simulink model "lab4"  (R2016b)
settings: Solver=VariableStepAuto  StartTime=0.0  StopTime=totaltime  RelTol=1e-3
undefined symbols (not defined in the file or in its folder): h, st
libraries: xbsIndex_r4 x1191
(part 1 of 3)
settings Model: Creator=rm101  LastModifiedBy=rm101

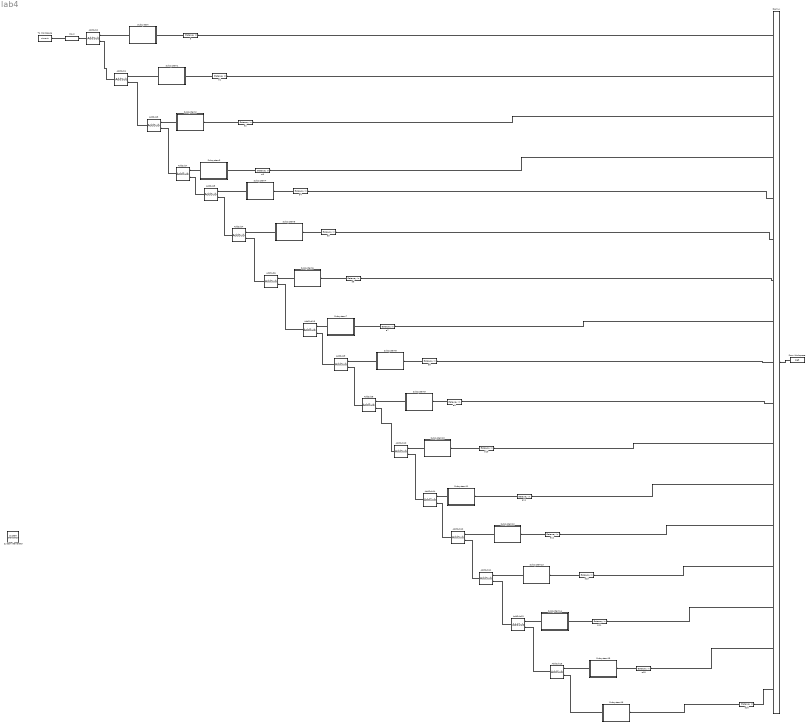
== system lab4 ==
  " System Generator" : xbsIndex_r4/ System Generator  Tag=genX  xilinxfamily=zynq  part=xc7z020  speed=-1  package=clg484  synthesis_tool=Vivado  clock_wrapper=Clock Enables  directory=E:/YG/generator/5_3  proj_type=Vivado  Synth_file=Vivado Synthesis Defaults  Impl_file=Vivado Implementation Defaults  testbench=off  simulink_period=st  sysclk_period=st*10e8  dcm_input_clock_period=10  incr_netlist=off  trim_vbits=Everywhere in SubSystem  dbl_ovrd=According to Block Masks  core_generation=According to Block Masks  run_coregen=off  deprecated_control=off  eval_field=0  block_type=sysgen
  AddSub{1..16} (16 alike) : xbsIndex_r4/AddSub  mode=Addition  use_carryin=off  use_carryout=off  en=off  latency=0  precision=User Defined  arith_type="Signed  (2's comp)"  n_bits=17  bin_pt=14  quantization=Truncate  overflow=Wrap  use_behavioral_HDL=off  hw_selection=Fabric  pipelined=off  dbl_ovrd=off  block_type=addsub
  Demux : Demux  Outputs=17
  Dout : xbsIndex_r4/Gateway Out  inherit_from_input=off  hdl_port=on  rows=1  columns=1  UseAsDAC=off  DACChannel='1'  interface=None  automatic_assignment=on  address_offset=hex2dec('00')  intf_name=''  intf_description=''  timing_constraint=None  locs_specified=off  LOCs={}  io_standard={}  block_type=gatewayout
  From Workspace : FromWorkspace  VariableName=sig3  SampleTime=0  Interpolate=off  OutputAfterFinalValue=Holding final value
  Subsystem : Subsystem
  Subsystem1 : Subsystem
  Subsystem10 : Subsystem
  Subsystem11 : Subsystem
  Subsystem12 : Subsystem
  Subsystem13 : Subsystem
  Subsystem14 : Subsystem
  Subsystem15 : Subsystem
  Subsystem16 : Subsystem
  Subsystem2 : Subsystem
  Subsystem3 : Subsystem
  Subsystem4 : Subsystem
  Subsystem5 : Subsystem
  Subsystem6 : Subsystem
  Subsystem7 : Subsystem
  Subsystem8 : Subsystem
  Subsystem9 : Subsystem
  To Workspace : ToWorkspace  VariableName=simout  SaveFormat=Timeseries  SampleTime=-1
  a{,1..16} (17 alike) : xbsIndex_r4/Gateway In  gui_display_data_type=Fixed-point  arith_type="Signed  (2's comp)"  n_bits=8  bin_pt=6  preci_type=Single  exp_width=8  frac_width=24  rows=1  columns=1  quantization="Round  (unbiased: +/- Inf)"  overflow=Saturate  period=st  UseAsADC=off  ADCChannel='1'  interface=None  automatic_assignment=on  address_offset=hex2dec('00')  intf_name=''  intf_description=''  default_value=0  timing_constraint=None  locs_specified=off  LOCs={}  io_standard={}  inherit_from_input=off  hdl_port=on  dbl_ovrd=off  block_type=gatewayin
  wires:
  Dout/1 -> To Workspace/1
  AddSub2/1 -> Dout/1
  Subsystem/1(Out1) -> AddSub2/1
  AddSub1/1 -> AddSub2/2
  Subsystem1/1(Out1) -> AddSub1/1
  AddSub3/1 -> AddSub1/2
  Subsystem2/1(Out1) -> AddSub3/1
  AddSub7/1 -> AddSub3/2
  AddSub5/1 -> AddSub7/2
  Subsystem4/1(Out1) -> AddSub5/1
  AddSub4/1 -> AddSub5/2
  Subsystem5/1(Out1) -> AddSub4/1
  AddSub6/1 -> AddSub4/2
  Subsystem6/1(Out1) -> AddSub6/1
  AddSub15/1 -> AddSub6/2
  Subsystem3/1(Out1) -> AddSub7/1
  Subsystem8/1(Out1) -> AddSub9/1
  AddSub8/1 -> AddSub9/2
  Subsystem9/1(Out1) -> AddSub8/1
  AddSub10/1 -> AddSub8/2
  Subsystem10/1(Out1) -> AddSub10/1
  AddSub14/1 -> AddSub10/2
  AddSub12/1 -> AddSub14/2
  Subsystem12/1(Out1) -> AddSub12/1
  AddSub11/1 -> AddSub12/2
  Subsystem13/1(Out1) -> AddSub11/1
  AddSub13/1 -> AddSub11/2
  Subsystem14/1(Out1) -> AddSub13/1
  AddSub16/1 -> AddSub13/2
  Subsystem11/1(Out1) -> AddSub14/1
  Subsystem7/1(Out1) -> AddSub15/1
  AddSub9/1 -> AddSub15/2
  Subsystem15/1(Out1) -> AddSub16/1
  Subsystem16/1(Out1) -> AddSub16/2
  From Workspace/1 -> Demux/1
  Demux/2 -> a1/1
  Demux/3 -> a2/1
  Demux/4 -> a3/1
  Demux/5 -> a4/1
  Demux/6 -> a5/1
  Demux/7 -> a6/1
  Demux/8 -> a7/1
  Demux/9 -> a8/1
  Demux/10 -> a9/1
  Demux/11 -> a10/1
  Demux/12 -> a11/1
  Demux/13 -> a12/1
  Demux/14 -> a13/1
  Demux/15 -> a14/1
  Demux/16 -> a15/1
  Demux/17 -> a16/1
  Demux/1 -> a/1
  a/1 -> Subsystem/1(In1)
  a1/1 -> Subsystem1/1(In1)
  a3/1 -> Subsystem3/1(In1)
  a2/1 -> Subsystem2/1(In1)
  a4/1 -> Subsystem4/1(In1)
  a5/1 -> Subsystem5/1(In1)
  a6/1 -> Subsystem6/1(In1)
  a7/1 -> Subsystem7/1(In1)
  a8/1 -> Subsystem8/1(In1)
  a9/1 -> Subsystem9/1(In1)
  a10/1 -> Subsystem10/1(In1)
  a11/1 -> Subsystem11/1(In1)
  a12/1 -> Subsystem12/1(In1)
  a13/1 -> Subsystem13/1(In1)
  a14/1 -> Subsystem14/1(In1)
  a15/1 -> Subsystem15/1(In1)
  a16/1 -> Subsystem16/1(In1)

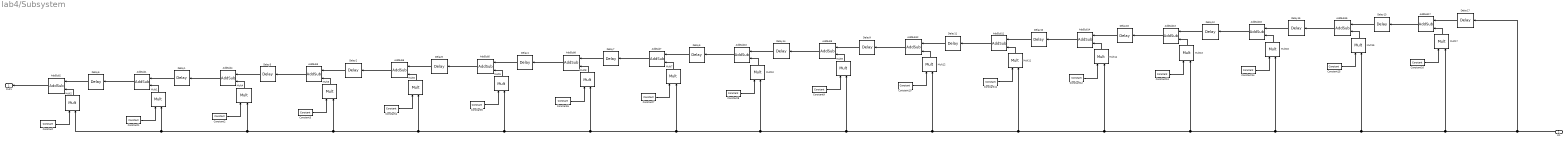
== system lab4/Subsystem ==
  In1 : Inport
  AddSub{1..17} (17 alike) : xbsIndex_r4/AddSub  mode=Addition  use_carryin=off  use_carryout=off  en=off  latency=0  precision=User Defined  arith_type="Signed  (2's comp)"  n_bits=17  bin_pt=14  quantization=Truncate  overflow=Wrap  use_behavioral_HDL=off  hw_selection=Fabric  pipelined=off  dbl_ovrd=off  block_type=addsub
  Constant : xbsIndex_r4/Constant  const=h(17,17)  gui_display_data_type=Fixed-point  arith_type=Signed (2's comp)  n_bits=16  bin_pt=14  preci_type=Single  exp_width=8  frac_width=24  explicit_period=off  period=1  equ=P=C  opselect=C  inp2=PCIN>>17  opr=+  inp1=P  carry=CIN  dbl_ovrd=off  block_type=constant
  Constant1 : xbsIndex_r4/Constant  const=h(17,16)  gui_display_data_type=Fixed-point  arith_type=Signed (2's comp)  n_bits=16  bin_pt=14  preci_type=Single  exp_width=8  frac_width=24  explicit_period=off  period=1  equ=P=C  opselect=C  inp2=PCIN>>17  opr=+  inp1=P  carry=CIN  dbl_ovrd=off  block_type=constant
  Constant10 : xbsIndex_r4/Constant  const=h(17,7)  gui_display_data_type=Fixed-point  arith_type=Signed (2's comp)  n_bits=16  bin_pt=14  preci_type=Single  exp_width=8  frac_width=24  explicit_period=off  period=1  equ=P=C  opselect=C  inp2=PCIN>>17  opr=+  inp1=P  carry=CIN  dbl_ovrd=off  block_type=constant
  Constant11 : xbsIndex_r4/Constant  const=h(17,6)  gui_display_data_type=Fixed-point  arith_type=Signed (2's comp)  n_bits=16  bin_pt=14  preci_type=Single  exp_width=8  frac_width=24  explicit_period=off  period=1  equ=P=C  opselect=C  inp2=PCIN>>17  opr=+  inp1=P  carry=CIN  dbl_ovrd=off  block_type=constant
  Constant12 : xbsIndex_r4/Constant  const=h(17,5)  gui_display_data_type=Fixed-point  arith_type=Signed (2's comp)  n_bits=16  bin_pt=14  preci_type=Single  exp_width=8  frac_width=24  explicit_period=off  period=1  equ=P=C  opselect=C  inp2=PCIN>>17  opr=+  inp1=P  carry=CIN  dbl_ovrd=off  block_type=constant
  Constant13 : xbsIndex_r4/Constant  const=h(17,4)  gui_display_data_type=Fixed-point  arith_type=Signed (2's comp)  n_bits=16  bin_pt=14  preci_type=Single  exp_width=8  frac_width=24  explicit_period=off  period=1  equ=P=C  opselect=C  inp2=PCIN>>17  opr=+  inp1=P  carry=CIN  dbl_ovrd=off  block_type=constant
  Constant14 : xbsIndex_r4/Constant  const=h(17,3)  gui_display_data_type=Fixed-point  arith_type=Signed (2's comp)  n_bits=16  bin_pt=14  preci_type=Single  exp_width=8  frac_width=24  explicit_period=off  period=1  equ=P=C  opselect=C  inp2=PCIN>>17  opr=+  inp1=P  carry=CIN  dbl_ovrd=off  block_type=constant
  Constant15 : xbsIndex_r4/Constant  const=h(17,2)  gui_display_data_type=Fixed-point  arith_type=Signed (2's comp)  n_bits=16  bin_pt=14  preci_type=Single  exp_width=8  frac_width=24  explicit_period=off  period=1  equ=P=C  opselect=C  inp2=PCIN>>17  opr=+  inp1=P  carry=CIN  dbl_ovrd=off  block_type=constant
  Constant16 : xbsIndex_r4/Constant  const=h(17,1)  gui_display_data_type=Fixed-point  arith_type=Signed (2's comp)  n_bits=17  bin_pt=14  preci_type=Single  exp_width=8  frac_width=24  explicit_period=off  period=1  equ=P=C  opselect=C  inp2=PCIN>>17  opr=+  inp1=P  carry=CIN  dbl_ovrd=off  block_type=constant
  Constant2 : xbsIndex_r4/Constant  const=h(17,15)  gui_display_data_type=Fixed-point  arith_type=Signed (2's comp)  n_bits=16  bin_pt=14  preci_type=Single  exp_width=8  frac_width=24  explicit_period=off  period=1  equ=P=C  opselect=C  inp2=PCIN>>17  opr=+  inp1=P  carry=CIN  dbl_ovrd=off  block_type=constant
  Constant3 : xbsIndex_r4/Constant  const=h(17,14)  gui_display_data_type=Fixed-point  arith_type=Signed (2's comp)  n_bits=16  bin_pt=14  preci_type=Single  exp_width=8  frac_width=24  explicit_period=off  period=1  equ=P=C  opselect=C  inp2=PCIN>>17  opr=+  inp1=P  carry=CIN  dbl_ovrd=off  block_type=constant
  Constant4 : xbsIndex_r4/Constant  const=h(17,13)  gui_display_data_type=Fixed-point  arith_type=Signed (2's comp)  n_bits=16  bin_pt=14  preci_type=Single  exp_width=8  frac_width=24  explicit_period=off  period=1  equ=P=C  opselect=C  inp2=PCIN>>17  opr=+  inp1=P  carry=CIN  dbl_ovrd=off  block_type=constant
  Constant5 : xbsIndex_r4/Constant  const=h(17,12)  gui_display_data_type=Fixed-point  arith_type=Signed (2's comp)  n_bits=16  bin_pt=14  preci_type=Single  exp_width=8  frac_width=24  explicit_period=off  period=1  equ=P=C  opselect=C  inp2=PCIN>>17  opr=+  inp1=P  carry=CIN  dbl_ovrd=off  block_type=constant
  Constant6 : xbsIndex_r4/Constant  const=h(17,11)  gui_display_data_type=Fixed-point  arith_type=Signed (2's comp)  n_bits=16  bin_pt=14  preci_type=Single  exp_width=8  frac_width=24  explicit_period=off  period=1  equ=P=C  opselect=C  inp2=PCIN>>17  opr=+  inp1=P  carry=CIN  dbl_ovrd=off  block_type=constant
  Constant7 : xbsIndex_r4/Constant  const=h(17,10)  gui_display_data_type=Fixed-point  arith_type=Signed (2's comp)  n_bits=16  bin_pt=14  preci_type=Single  exp_width=8  frac_width=24  explicit_period=off  period=1  equ=P=C  opselect=C  inp2=PCIN>>17  opr=+  inp1=P  carry=CIN  dbl_ovrd=off  block_type=constant
  Constant8 : xbsIndex_r4/Constant  const=h(17,9)  gui_display_data_type=Fixed-point  arith_type=Signed (2's comp)  n_bits=16  bin_pt=14  preci_type=Single  exp_width=8  frac_width=24  explicit_period=off  period=1  equ=P=C  opselect=C  inp2=PCIN>>17  opr=+  inp1=P  carry=CIN  dbl_ovrd=off  block_type=constant
  Constant9 : xbsIndex_r4/Constant  const=h(17,8)  gui_display_data_type=Fixed-point  arith_type=Signed (2's comp)  n_bits=16  bin_pt=14  preci_type=Single  exp_width=8  frac_width=24  explicit_period=off  period=1  equ=P=C  opselect=C  inp2=PCIN>>17  opr=+  inp1=P  carry=CIN  dbl_ovrd=off  block_type=constant
  Delay{1..17} (17 alike) : xbsIndex_r4/Delay  rst=off  infoeditControl=Selection of Reset will increase slice count due to use of real FFs and instead of SRLs  en=off  latency=1  reg_retiming=off  dbl_ovrd=off  block_type=delay
  Mult{1..17} (17 alike) : xbsIndex_r4/Mult  precision=User Defined  arith_type="Signed  (2's comp)"  n_bits=16  bin_pt=14  quantization="Round  (unbiased: +/- Inf)"  overflow=Flag as error  en=off  latency=0  use_behavioral_HDL=off  opt=Speed  use_embedded=on  optimum_pipeline=off  pipeline=on  dbl_ovrd=off  use_rpm=on  placement_style=Triangular  block_type=mult
  Out1 : Outport
  wires:
  Mult2/1 -> AddSub2/2
  AddSub2/1 -> Out1/1
  Delay6/1 -> AddSub2/1
  Constant2/1 -> Mult4/1
  AddSub4/1 -> Delay1/1
  Mult4/1 -> AddSub4/2
  Delay3/1 -> AddSub4/1
  Constant4/1 -> Mult6/1
  AddSub12/1 -> Delay9/1
  Constant3/1 -> Mult3/1
  Mult13/1 -> AddSub13/2
  AddSub13/1 -> Delay16/1
  Delay7/1 -> AddSub8/1
  Constant13/1 -> Mult13/1
  Mult3/1 -> AddSub3/2
  Mult8/1 -> AddSub8/2
  Delay8/1 -> AddSub6/1
  Delay2/1 -> AddSub3/1
  AddSub3/1 -> Delay3/1
  Delay14/1 -> AddSub10/1
  AddSub11/1 -> Delay11/1
  AddSub9/1 -> Delay14/1
  AddSub6/1 -> Delay2/1
  Delay5/1 -> AddSub7/1
  Constant7/1 -> Mult7/1
  Mult5/1 -> AddSub5/2
  Constant5/1 -> Mult5/1
  Mult12/1 -> AddSub12/2
  Mult7/1 -> AddSub7/2
  AddSub7/1 -> Delay7/1
  Delay11/1 -> AddSub12/1
  Mult11/1 -> AddSub11/2
  AddSub8/1 -> Delay4/1
  Delay4/1 -> AddSub5/1
  Constant6/1 -> Mult8/1
  Mult6/1 -> AddSub6/2
  AddSub5/1 -> Delay8/1
  Delay15/1 -> AddSub16/1
  AddSub10/1 -> Delay5/1
  Delay9/1 -> AddSub9/1
  Mult10/1 -> AddSub10/2
  Delay16/1 -> AddSub14/1
  Delay13/1 -> AddSub15/1
  Mult9/1 -> AddSub9/2
  Constant8/1 -> Mult10/1
  Constant15/1 -> Mult15/1
  Constant12/1 -> Mult14/1
  Delay10/1 -> AddSub11/1
  Delay12/1 -> AddSub13/1
  AddSub16/1 -> Delay12/1
  Mult15/1 -> AddSub15/2
  AddSub14/1 -> Delay10/1
  Mult16/1 -> AddSub16/2
  Mult14/1 -> AddSub14/2
  Constant11/1 -> Mult11/1
  Constant9/1 -> Mult9/1
  AddSub15/1 -> Delay15/1
  Constant10/1 -> Mult12/1
  Constant14/1 -> Mult16/1
  In1/1 -> Delay17/1, Mult17/2, Mult15/2, Mult16/2, Mult13/2, Mult14/2, Mult11/2, Mult12/2, Mult9/2, Mult10/2, Mult7/2, Mult8/2, Mult5/2, Mult6/2, Mult3/2, Mult4/2, Mult2/2, Mult1/2
  Delay17/1 -> AddSub17/1
  AddSub17/1 -> Delay13/1
  Mult17/1 -> AddSub17/2
  Constant16/1 -> Mult17/1
  Constant/1 -> Mult2/1
  Delay1/1 -> AddSub1/1
  Mult1/1 -> AddSub1/2
  Constant1/1 -> Mult1/1
  AddSub1/1 -> Delay6/1

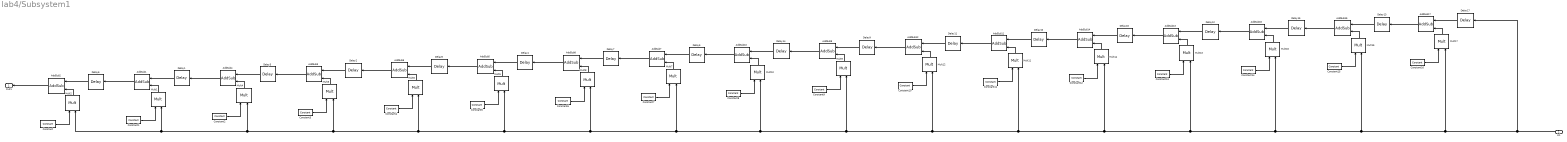
== system lab4/Subsystem1 ==
  In1 : Inport
  AddSub{1..17} (17 alike) : xbsIndex_r4/AddSub  mode=Addition  use_carryin=off  use_carryout=off  en=off  latency=0  precision=User Defined  arith_type="Signed  (2's comp)"  n_bits=17  bin_pt=14  quantization=Truncate  overflow=Wrap  use_behavioral_HDL=off  hw_selection=Fabric  pipelined=off  dbl_ovrd=off  block_type=addsub
  Constant : xbsIndex_r4/Constant  const=h(16,17)  gui_display_data_type=Fixed-point  arith_type=Signed (2's comp)  n_bits=16  bin_pt=14  preci_type=Single  exp_width=8  frac_width=24  explicit_period=off  period=1  equ=P=C  opselect=C  inp2=PCIN>>17  opr=+  inp1=P  carry=CIN  dbl_ovrd=off  block_type=constant
  Constant1 : xbsIndex_r4/Constant  const=h(16,16)  gui_display_data_type=Fixed-point  arith_type=Signed (2's comp)  n_bits=16  bin_pt=14  preci_type=Single  exp_width=8  frac_width=24  explicit_period=off  period=1  equ=P=C  opselect=C  inp2=PCIN>>17  opr=+  inp1=P  carry=CIN  dbl_ovrd=off  block_type=constant
  Constant10 : xbsIndex_r4/Constant  const=h(16,7)  gui_display_data_type=Fixed-point  arith_type=Signed (2's comp)  n_bits=16  bin_pt=14  preci_type=Single  exp_width=8  frac_width=24  explicit_period=off  period=1  equ=P=C  opselect=C  inp2=PCIN>>17  opr=+  inp1=P  carry=CIN  dbl_ovrd=off  block_type=constant
  Constant11 : xbsIndex_r4/Constant  const=h(16,6)  gui_display_data_type=Fixed-point  arith_type=Signed (2's comp)  n_bits=16  bin_pt=14  preci_type=Single  exp_width=8  frac_width=24  explicit_period=off  period=1  equ=P=C  opselect=C  inp2=PCIN>>17  opr=+  inp1=P  carry=CIN  dbl_ovrd=off  block_type=constant
  Constant12 : xbsIndex_r4/Constant  const=h(16,5)  gui_display_data_type=Fixed-point  arith_type=Signed (2's comp)  n_bits=16  bin_pt=14  preci_type=Single  exp_width=8  frac_width=24  explicit_period=off  period=1  equ=P=C  opselect=C  inp2=PCIN>>17  opr=+  inp1=P  carry=CIN  dbl_ovrd=off  block_type=constant
  Constant13 : xbsIndex_r4/Constant  const=h(16,4)  gui_display_data_type=Fixed-point  arith_type=Signed (2's comp)  n_bits=16  bin_pt=14  preci_type=Single  exp_width=8  frac_width=24  explicit_period=off  period=1  equ=P=C  opselect=C  inp2=PCIN>>17  opr=+  inp1=P  carry=CIN  dbl_ovrd=off  block_type=constant
  Constant14 : xbsIndex_r4/Constant  const=h(16,3)  gui_display_data_type=Fixed-point  arith_type=Signed (2's comp)  n_bits=16  bin_pt=14  preci_type=Single  exp_width=8  frac_width=24  explicit_period=off  period=1  equ=P=C  opselect=C  inp2=PCIN>>17  opr=+  inp1=P  carry=CIN  dbl_ovrd=off  block_type=constant
  Constant15 : xbsIndex_r4/Constant  const=h(16,2)  gui_display_data_type=Fixed-point  arith_type=Signed (2's comp)  n_bits=16  bin_pt=14  preci_type=Single  exp_width=8  frac_width=24  explicit_period=off  period=1  equ=P=C  opselect=C  inp2=PCIN>>17  opr=+  inp1=P  carry=CIN  dbl_ovrd=off  block_type=constant
  Constant16 : xbsIndex_r4/Constant  const=h(16,1)  gui_display_data_type=Fixed-point  arith_type=Signed (2's comp)  n_bits=17  bin_pt=14  preci_type=Single  exp_width=8  frac_width=24  explicit_period=off  period=1  equ=P=C  opselect=C  inp2=PCIN>>17  opr=+  inp1=P  carry=CIN  dbl_ovrd=off  block_type=constant
  Constant2 : xbsIndex_r4/Constant  const=h(16,15)  gui_display_data_type=Fixed-point  arith_type=Signed (2's comp)  n_bits=16  bin_pt=14  preci_type=Single  exp_width=8  frac_width=24  explicit_period=off  period=1  equ=P=C  opselect=C  inp2=PCIN>>17  opr=+  inp1=P  carry=CIN  dbl_ovrd=off  block_type=constant
  Constant3 : xbsIndex_r4/Constant  const=h(16,14)  gui_display_data_type=Fixed-point  arith_type=Signed (2's comp)  n_bits=16  bin_pt=14  preci_type=Single  exp_width=8  frac_width=24  explicit_period=off  period=1  equ=P=C  opselect=C  inp2=PCIN>>17  opr=+  inp1=P  carry=CIN  dbl_ovrd=off  block_type=constant
  Constant4 : xbsIndex_r4/Constant  const=h(16,13)  gui_display_data_type=Fixed-point  arith_type=Signed (2's comp)  n_bits=16  bin_pt=14  preci_type=Single  exp_width=8  frac_width=24  explicit_period=off  period=1  equ=P=C  opselect=C  inp2=PCIN>>17  opr=+  inp1=P  carry=CIN  dbl_ovrd=off  block_type=constant
  Constant5 : xbsIndex_r4/Constant  const=h(16,12)  gui_display_data_type=Fixed-point  arith_type=Signed (2's comp)  n_bits=16  bin_pt=14  preci_type=Single  exp_width=8  frac_width=24  explicit_period=off  period=1  equ=P=C  opselect=C  inp2=PCIN>>17  opr=+  inp1=P  carry=CIN  dbl_ovrd=off  block_type=constant
  Constant6 : xbsIndex_r4/Constant  const=h(16,11)  gui_display_data_type=Fixed-point  arith_type=Signed (2's comp)  n_bits=16  bin_pt=14  preci_type=Single  exp_width=8  frac_width=24  explicit_period=off  period=1  equ=P=C  opselect=C  inp2=PCIN>>17  opr=+  inp1=P  carry=CIN  dbl_ovrd=off  block_type=constant
  Constant7 : xbsIndex_r4/Constant  const=h(16,10)  gui_display_data_type=Fixed-point  arith_type=Signed (2's comp)  n_bits=16  bin_pt=14  preci_type=Single  exp_width=8  frac_width=24  explicit_period=off  period=1  equ=P=C  opselect=C  inp2=PCIN>>17  opr=+  inp1=P  carry=CIN  dbl_ovrd=off  block_type=constant
  Constant8 : xbsIndex_r4/Constant  const=h(16,9)  gui_display_data_type=Fixed-point  arith_type=Signed (2's comp)  n_bits=16  bin_pt=14  preci_type=Single  exp_width=8  frac_width=24  explicit_period=off  period=1  equ=P=C  opselect=C  inp2=PCIN>>17  opr=+  inp1=P  carry=CIN  dbl_ovrd=off  block_type=constant
  Constant9 : xbsIndex_r4/Constant  const=h(16,8)  gui_display_data_type=Fixed-point  arith_type=Signed (2's comp)  n_bits=16  bin_pt=14  preci_type=Single  exp_width=8  frac_width=24  explicit_period=off  period=1  equ=P=C  opselect=C  inp2=PCIN>>17  opr=+  inp1=P  carry=CIN  dbl_ovrd=off  block_type=constant
  Delay{1..17} (17 alike) : xbsIndex_r4/Delay  rst=off  infoeditControl=Selection of Reset will increase slice count due to use of real FFs and instead of SRLs  en=off  latency=1  reg_retiming=off  dbl_ovrd=off  block_type=delay
  Mult{1..17} (17 alike) : xbsIndex_r4/Mult  precision=User Defined  arith_type="Signed  (2's comp)"  n_bits=16  bin_pt=14  quantization="Round  (unbiased: +/- Inf)"  overflow=Flag as error  en=off  latency=0  use_behavioral_HDL=off  opt=Speed  use_embedded=on  optimum_pipeline=off  pipeline=on  dbl_ovrd=off  use_rpm=on  placement_style=Triangular  block_type=mult
  Out1 : Outport
  wires:
  Mult2/1 -> AddSub2/2
  AddSub2/1 -> Out1/1
  Delay6/1 -> AddSub2/1
  Constant2/1 -> Mult4/1
  AddSub4/1 -> Delay1/1
  Mult4/1 -> AddSub4/2
  Delay3/1 -> AddSub4/1
  Constant4/1 -> Mult6/1
  AddSub12/1 -> Delay9/1
  Constant3/1 -> Mult3/1
  Mult13/1 -> AddSub13/2
  AddSub13/1 -> Delay16/1
  Delay7/1 -> AddSub8/1
  Constant13/1 -> Mult13/1
  Mult3/1 -> AddSub3/2
  Mult8/1 -> AddSub8/2
  Delay8/1 -> AddSub6/1
  Delay2/1 -> AddSub3/1
  AddSub3/1 -> Delay3/1
  Delay14/1 -> AddSub10/1
  AddSub11/1 -> Delay11/1
  AddSub9/1 -> Delay14/1
  AddSub6/1 -> Delay2/1
  Delay5/1 -> AddSub7/1
  Constant7/1 -> Mult7/1
  Mult5/1 -> AddSub5/2
  Constant5/1 -> Mult5/1
  Mult12/1 -> AddSub12/2
  Mult7/1 -> AddSub7/2
  AddSub7/1 -> Delay7/1
  Delay11/1 -> AddSub12/1
  Mult11/1 -> AddSub11/2
  AddSub8/1 -> Delay4/1
  Delay4/1 -> AddSub5/1
  Constant6/1 -> Mult8/1
  Mult6/1 -> AddSub6/2
  AddSub5/1 -> Delay8/1
  Delay15/1 -> AddSub16/1
  AddSub10/1 -> Delay5/1
  Delay9/1 -> AddSub9/1
  Mult10/1 -> AddSub10/2
  Delay16/1 -> AddSub14/1
  Delay13/1 -> AddSub15/1
  Mult9/1 -> AddSub9/2
  Constant8/1 -> Mult10/1
  Constant15/1 -> Mult15/1
  Constant12/1 -> Mult14/1
  Delay10/1 -> AddSub11/1
  Delay12/1 -> AddSub13/1
  AddSub16/1 -> Delay12/1
  Mult15/1 -> AddSub15/2
  AddSub14/1 -> Delay10/1
  Mult16/1 -> AddSub16/2
  Mult14/1 -> AddSub14/2
  Constant11/1 -> Mult11/1
  Constant9/1 -> Mult9/1
  AddSub15/1 -> Delay15/1
  Constant10/1 -> Mult12/1
  Constant14/1 -> Mult16/1
  In1/1 -> Delay17/1, Mult17/2, Mult15/2, Mult16/2, Mult13/2, Mult14/2, Mult11/2, Mult12/2, Mult9/2, Mult10/2, Mult7/2, Mult8/2, Mult5/2, Mult6/2, Mult3/2, Mult4/2, Mult2/2, Mult1/2
  Delay17/1 -> AddSub17/1
  AddSub17/1 -> Delay13/1
  Mult17/1 -> AddSub17/2
  Constant16/1 -> Mult17/1
  Constant/1 -> Mult2/1
  Delay1/1 -> AddSub1/1
  Mult1/1 -> AddSub1/2
  Constant1/1 -> Mult1/1
  AddSub1/1 -> Delay6/1

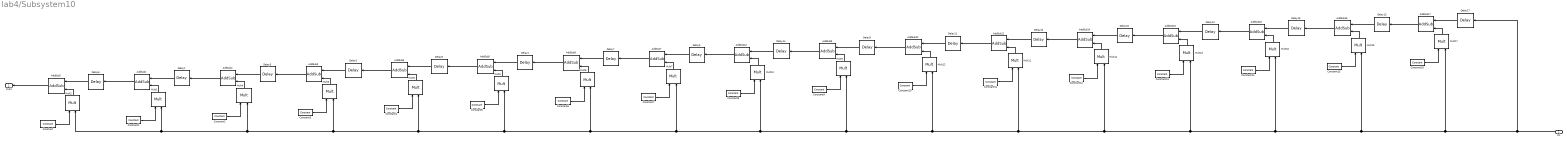
== system lab4/Subsystem10 ==
  In1 : Inport
  AddSub{1..17} (17 alike) : xbsIndex_r4/AddSub  mode=Addition  use_carryin=off  use_carryout=off  en=off  latency=0  precision=User Defined  arith_type="Signed  (2's comp)"  n_bits=17  bin_pt=14  quantization=Truncate  overflow=Wrap  use_behavioral_HDL=off  hw_selection=Fabric  pipelined=off  dbl_ovrd=off  block_type=addsub
  Constant : xbsIndex_r4/Constant  const=h(7,17)  gui_display_data_type=Fixed-point  arith_type=Signed (2's comp)  n_bits=16  bin_pt=14  preci_type=Single  exp_width=8  frac_width=24  explicit_period=off  period=1  equ=P=C  opselect=C  inp2=PCIN>>17  opr=+  inp1=P  carry=CIN  dbl_ovrd=off  block_type=constant
  Constant1 : xbsIndex_r4/Constant  const=h(7,16)  gui_display_data_type=Fixed-point  arith_type=Signed (2's comp)  n_bits=16  bin_pt=14  preci_type=Single  exp_width=8  frac_width=24  explicit_period=off  period=1  equ=P=C  opselect=C  inp2=PCIN>>17  opr=+  inp1=P  carry=CIN  dbl_ovrd=off  block_type=constant
  Constant10 : xbsIndex_r4/Constant  const=h(7,7)  gui_display_data_type=Fixed-point  arith_type=Signed (2's comp)  n_bits=16  bin_pt=14  preci_type=Single  exp_width=8  frac_width=24  explicit_period=off  period=1  equ=P=C  opselect=C  inp2=PCIN>>17  opr=+  inp1=P  carry=CIN  dbl_ovrd=off  block_type=constant
  Constant11 : xbsIndex_r4/Constant  const=h(7,6)  gui_display_data_type=Fixed-point  arith_type=Signed (2's comp)  n_bits=16  bin_pt=14  preci_type=Single  exp_width=8  frac_width=24  explicit_period=off  period=1  equ=P=C  opselect=C  inp2=PCIN>>17  opr=+  inp1=P  carry=CIN  dbl_ovrd=off  block_type=constant
  Constant12 : xbsIndex_r4/Constant  const=h(7,5)  gui_display_data_type=Fixed-point  arith_type=Signed (2's comp)  n_bits=16  bin_pt=14  preci_type=Single  exp_width=8  frac_width=24  explicit_period=off  period=1  equ=P=C  opselect=C  inp2=PCIN>>17  opr=+  inp1=P  carry=CIN  dbl_ovrd=off  block_type=constant
  Constant13 : xbsIndex_r4/Constant  const=h(7,4)  gui_display_data_type=Fixed-point  arith_type=Signed (2's comp)  n_bits=16  bin_pt=14  preci_type=Single  exp_width=8  frac_width=24  explicit_period=off  period=1  equ=P=C  opselect=C  inp2=PCIN>>17  opr=+  inp1=P  carry=CIN  dbl_ovrd=off  block_type=constant
  Constant14 : xbsIndex_r4/Constant  const=h(7,3)  gui_display_data_type=Fixed-point  arith_type=Signed (2's comp)  n_bits=16  bin_pt=14  preci_type=Single  exp_width=8  frac_width=24  explicit_period=off  period=1  equ=P=C  opselect=C  inp2=PCIN>>17  opr=+  inp1=P  carry=CIN  dbl_ovrd=off  block_type=constant
  Constant15 : xbsIndex_r4/Constant  const=h(7,2)  gui_display_data_type=Fixed-point  arith_type=Signed (2's comp)  n_bits=16  bin_pt=14  preci_type=Single  exp_width=8  frac_width=24  explicit_period=off  period=1  equ=P=C  opselect=C  inp2=PCIN>>17  opr=+  inp1=P  carry=CIN  dbl_ovrd=off  block_type=constant
  Constant16 : xbsIndex_r4/Constant  const=h(7,1)  gui_display_data_type=Fixed-point  arith_type=Signed (2's comp)  n_bits=17  bin_pt=14  preci_type=Single  exp_width=8  frac_width=24  explicit_period=off  period=1  equ=P=C  opselect=C  inp2=PCIN>>17  opr=+  inp1=P  carry=CIN  dbl_ovrd=off  block_type=constant
  Constant2 : xbsIndex_r4/Constant  const=h(7,15)  gui_display_data_type=Fixed-point  arith_type=Signed (2's comp)  n_bits=16  bin_pt=14  preci_type=Single  exp_width=8  frac_width=24  explicit_period=off  period=1  equ=P=C  opselect=C  inp2=PCIN>>17  opr=+  inp1=P  carry=CIN  dbl_ovrd=off  block_type=constant
  Constant3 : xbsIndex_r4/Constant  const=h(7,14)  gui_display_data_type=Fixed-point  arith_type=Signed (2's comp)  n_bits=16  bin_pt=14  preci_type=Single  exp_width=8  frac_width=24  explicit_period=off  period=1  equ=P=C  opselect=C  inp2=PCIN>>17  opr=+  inp1=P  carry=CIN  dbl_ovrd=off  block_type=constant
  Constant4 : xbsIndex_r4/Constant  const=h(7,13)  gui_display_data_type=Fixed-point  arith_type=Signed (2's comp)  n_bits=16  bin_pt=14  preci_type=Single  exp_width=8  frac_width=24  explicit_period=off  period=1  equ=P=C  opselect=C  inp2=PCIN>>17  opr=+  inp1=P  carry=CIN  dbl_ovrd=off  block_type=constant
  Constant5 : xbsIndex_r4/Constant  const=h(7,12)  gui_display_data_type=Fixed-point  arith_type=Signed (2's comp)  n_bits=16  bin_pt=14  preci_type=Single  exp_width=8  frac_width=24  explicit_period=off  period=1  equ=P=C  opselect=C  inp2=PCIN>>17  opr=+  inp1=P  carry=CIN  dbl_ovrd=off  block_type=constant
  Constant6 : xbsIndex_r4/Constant  const=h(7,11)  gui_display_data_type=Fixed-point  arith_type=Signed (2's comp)  n_bits=16  bin_pt=14  preci_type=Single  exp_width=8  frac_width=24  explicit_period=off  period=1  equ=P=C  opselect=C  inp2=PCIN>>17  opr=+  inp1=P  carry=CIN  dbl_ovrd=off  block_type=constant
  Constant7 : xbsIndex_r4/Constant  const=h(7,10)  gui_display_data_type=Fixed-point  arith_type=Signed (2's comp)  n_bits=16  bin_pt=14  preci_type=Single  exp_width=8  frac_width=24  explicit_period=off  period=1  equ=P=C  opselect=C  inp2=PCIN>>17  opr=+  inp1=P  carry=CIN  dbl_ovrd=off  block_type=constant
  Constant8 : xbsIndex_r4/Constant  const=h(7,9)  gui_display_data_type=Fixed-point  arith_type=Signed (2's comp)  n_bits=16  bin_pt=14  preci_type=Single  exp_width=8  frac_width=24  explicit_period=off  period=1  equ=P=C  opselect=C  inp2=PCIN>>17  opr=+  inp1=P  carry=CIN  dbl_ovrd=off  block_type=constant
  Constant9 : xbsIndex_r4/Constant  const=h(7,8)  gui_display_data_type=Fixed-point  arith_type=Signed (2's comp)  n_bits=16  bin_pt=14  preci_type=Single  exp_width=8  frac_width=24  explicit_period=off  period=1  equ=P=C  opselect=C  inp2=PCIN>>17  opr=+  inp1=P  carry=CIN  dbl_ovrd=off  block_type=constant
  Delay{1..17} (17 alike) : xbsIndex_r4/Delay  rst=off  infoeditControl=Selection of Reset will increase slice count due to use of real FFs and instead of SRLs  en=off  latency=1  reg_retiming=off  dbl_ovrd=off  block_type=delay
  Mult{1..17} (17 alike) : xbsIndex_r4/Mult  precision=User Defined  arith_type="Signed  (2's comp)"  n_bits=16  bin_pt=14  quantization="Round  (unbiased: +/- Inf)"  overflow=Flag as error  en=off  latency=0  use_behavioral_HDL=off  opt=Speed  use_embedded=on  optimum_pipeline=off  pipeline=on  dbl_ovrd=off  use_rpm=on  placement_style=Triangular  block_type=mult
  Out1 : Outport
  wires:
  Mult2/1 -> AddSub2/2
  AddSub2/1 -> Out1/1
  Delay6/1 -> AddSub2/1
  Constant2/1 -> Mult4/1
  AddSub4/1 -> Delay1/1
  Mult4/1 -> AddSub4/2
  Delay3/1 -> AddSub4/1
  Constant4/1 -> Mult6/1
  AddSub12/1 -> Delay9/1
  Constant3/1 -> Mult3/1
  Mult13/1 -> AddSub13/2
  AddSub13/1 -> Delay16/1
  Delay7/1 -> AddSub8/1
  Constant13/1 -> Mult13/1
  Mult3/1 -> AddSub3/2
  Mult8/1 -> AddSub8/2
  Delay8/1 -> AddSub6/1
  Delay2/1 -> AddSub3/1
  AddSub3/1 -> Delay3/1
  Delay14/1 -> AddSub10/1
  AddSub11/1 -> Delay11/1
  AddSub9/1 -> Delay14/1
  AddSub6/1 -> Delay2/1
  Delay5/1 -> AddSub7/1
  Constant7/1 -> Mult7/1
  Mult5/1 -> AddSub5/2
  Constant5/1 -> Mult5/1
  Mult12/1 -> AddSub12/2
  Mult7/1 -> AddSub7/2
  AddSub7/1 -> Delay7/1
  Delay11/1 -> AddSub12/1
  Mult11/1 -> AddSub11/2
  AddSub8/1 -> Delay4/1
  Delay4/1 -> AddSub5/1
  Constant6/1 -> Mult8/1
  Mult6/1 -> AddSub6/2
  AddSub5/1 -> Delay8/1
  Delay15/1 -> AddSub16/1
  AddSub10/1 -> Delay5/1
  Delay9/1 -> AddSub9/1
  Mult10/1 -> AddSub10/2
  Delay16/1 -> AddSub14/1
  Delay13/1 -> AddSub15/1
  Mult9/1 -> AddSub9/2
  Constant8/1 -> Mult10/1
  Constant15/1 -> Mult15/1
  Constant12/1 -> Mult14/1
  Delay10/1 -> AddSub11/1
  Delay12/1 -> AddSub13/1
  AddSub16/1 -> Delay12/1
  Mult15/1 -> AddSub15/2
  AddSub14/1 -> Delay10/1
  Mult16/1 -> AddSub16/2
  Mult14/1 -> AddSub14/2
  Constant11/1 -> Mult11/1
  Constant9/1 -> Mult9/1
  AddSub15/1 -> Delay15/1
  Constant10/1 -> Mult12/1
  Constant14/1 -> Mult16/1
  In1/1 -> Delay17/1, Mult17/2, Mult15/2, Mult16/2, Mult13/2, Mult14/2, Mult11/2, Mult12/2, Mult9/2, Mult10/2, Mult7/2, Mult8/2, Mult5/2, Mult6/2, Mult3/2, Mult4/2, Mult2/2, Mult1/2
  Delay17/1 -> AddSub17/1
  AddSub17/1 -> Delay13/1
  Mult17/1 -> AddSub17/2
  Constant16/1 -> Mult17/1
  Constant/1 -> Mult2/1
  Delay1/1 -> AddSub1/1
  Mult1/1 -> AddSub1/2
  Constant1/1 -> Mult1/1
  AddSub1/1 -> Delay6/1

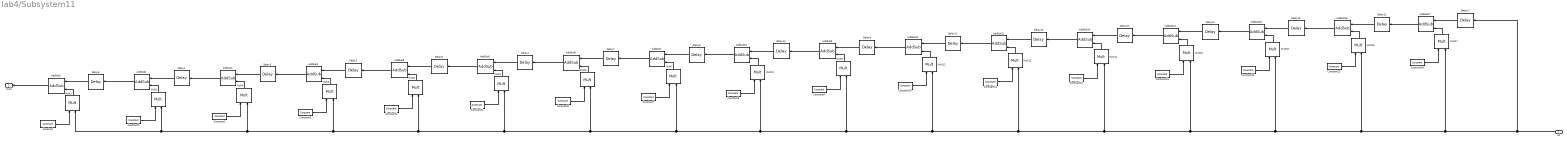
== system lab4/Subsystem11 ==
  In1 : Inport
  AddSub{1..17} (17 alike) : xbsIndex_r4/AddSub  mode=Addition  use_carryin=off  use_carryout=off  en=off  latency=0  precision=User Defined  arith_type="Signed  (2's comp)"  n_bits=17  bin_pt=14  quantization=Truncate  overflow=Wrap  use_behavioral_HDL=off  hw_selection=Fabric  pipelined=off  dbl_ovrd=off  block_type=addsub
  Constant : xbsIndex_r4/Constant  const=h(6,17)  gui_display_data_type=Fixed-point  arith_type=Signed (2's comp)  n_bits=16  bin_pt=14  preci_type=Single  exp_width=8  frac_width=24  explicit_period=off  period=1  equ=P=C  opselect=C  inp2=PCIN>>17  opr=+  inp1=P  carry=CIN  dbl_ovrd=off  block_type=constant
  Constant1 : xbsIndex_r4/Constant  const=h(6,16)  gui_display_data_type=Fixed-point  arith_type=Signed (2's comp)  n_bits=16  bin_pt=14  preci_type=Single  exp_width=8  frac_width=24  explicit_period=off  period=1  equ=P=C  opselect=C  inp2=PCIN>>17  opr=+  inp1=P  carry=CIN  dbl_ovrd=off  block_type=constant
  Constant10 : xbsIndex_r4/Constant  const=h(6,7)  gui_display_data_type=Fixed-point  arith_type=Signed (2's comp)  n_bits=16  bin_pt=14  preci_type=Single  exp_width=8  frac_width=24  explicit_period=off  period=1  equ=P=C  opselect=C  inp2=PCIN>>17  opr=+  inp1=P  carry=CIN  dbl_ovrd=off  block_type=constant
  Constant11 : xbsIndex_r4/Constant  const=h(6,6)  gui_display_data_type=Fixed-point  arith_type=Signed (2's comp)  n_bits=16  bin_pt=14  preci_type=Single  exp_width=8  frac_width=24  explicit_period=off  period=1  equ=P=C  opselect=C  inp2=PCIN>>17  opr=+  inp1=P  carry=CIN  dbl_ovrd=off  block_type=constant
  Constant12 : xbsIndex_r4/Constant  const=h(6,5)  gui_display_data_type=Fixed-point  arith_type=Signed (2's comp)  n_bits=16  bin_pt=14  preci_type=Single  exp_width=8  frac_width=24  explicit_period=off  period=1  equ=P=C  opselect=C  inp2=PCIN>>17  opr=+  inp1=P  carry=CIN  dbl_ovrd=off  block_type=constant
  Constant13 : xbsIndex_r4/Constant  const=h(6,4)  gui_display_data_type=Fixed-point  arith_type=Signed (2's comp)  n_bits=16  bin_pt=14  preci_type=Single  exp_width=8  frac_width=24  explicit_period=off  period=1  equ=P=C  opselect=C  inp2=PCIN>>17  opr=+  inp1=P  carry=CIN  dbl_ovrd=off  block_type=constant
  Constant14 : xbsIndex_r4/Constant  const=h(6,3)  gui_display_data_type=Fixed-point  arith_type=Signed (2's comp)  n_bits=16  bin_pt=14  preci_type=Single  exp_width=8  frac_width=24  explicit_period=off  period=1  equ=P=C  opselect=C  inp2=PCIN>>17  opr=+  inp1=P  carry=CIN  dbl_ovrd=off  block_type=constant
  Constant15 : xbsIndex_r4/Constant  const=h(6,2)  gui_display_data_type=Fixed-point  arith_type=Signed (2's comp)  n_bits=16  bin_pt=14  preci_type=Single  exp_width=8  frac_width=24  explicit_period=off  period=1  equ=P=C  opselect=C  inp2=PCIN>>17  opr=+  inp1=P  carry=CIN  dbl_ovrd=off  block_type=constant
  Constant16 : xbsIndex_r4/Constant  const=h(6,1)  gui_display_data_type=Fixed-point  arith_type=Signed (2's comp)  n_bits=17  bin_pt=14  preci_type=Single  exp_width=8  frac_width=24  explicit_period=off  period=1  equ=P=C  opselect=C  inp2=PCIN>>17  opr=+  inp1=P  carry=CIN  dbl_ovrd=off  block_type=constant
  Constant2 : xbsIndex_r4/Constant  const=h(6,15)  gui_display_data_type=Fixed-point  arith_type=Signed (2's comp)  n_bits=16  bin_pt=14  preci_type=Single  exp_width=8  frac_width=24  explicit_period=off  period=1  equ=P=C  opselect=C  inp2=PCIN>>17  opr=+  inp1=P  carry=CIN  dbl_ovrd=off  block_type=constant
  Constant3 : xbsIndex_r4/Constant  const=h(6,14)  gui_display_data_type=Fixed-point  arith_type=Signed (2's comp)  n_bits=16  bin_pt=14  preci_type=Single  exp_width=8  frac_width=24  explicit_period=off  period=1  equ=P=C  opselect=C  inp2=PCIN>>17  opr=+  inp1=P  carry=CIN  dbl_ovrd=off  block_type=constant
  Constant4 : xbsIndex_r4/Constant  const=h(6,13)  gui_display_data_type=Fixed-point  arith_type=Signed (2's comp)  n_bits=16  bin_pt=14  preci_type=Single  exp_width=8  frac_width=24  explicit_period=off  period=1  equ=P=C  opselect=C  inp2=PCIN>>17  opr=+  inp1=P  carry=CIN  dbl_ovrd=off  block_type=constant
  Constant5 : xbsIndex_r4/Constant  const=h(6,12)  gui_display_data_type=Fixed-point  arith_type=Signed (2's comp)  n_bits=16  bin_pt=14  preci_type=Single  exp_width=8  frac_width=24  explicit_period=off  period=1  equ=P=C  opselect=C  inp2=PCIN>>17  opr=+  inp1=P  carry=CIN  dbl_ovrd=off  block_type=constant
  Constant6 : xbsIndex_r4/Constant  const=h(6,11)  gui_display_data_type=Fixed-point  arith_type=Signed (2's comp)  n_bits=16  bin_pt=14  preci_type=Single  exp_width=8  frac_width=24  explicit_period=off  period=1  equ=P=C  opselect=C  inp2=PCIN>>17  opr=+  inp1=P  carry=CIN  dbl_ovrd=off  block_type=constant
  Constant7 : xbsIndex_r4/Constant  const=h(6,10)  gui_display_data_type=Fixed-point  arith_type=Signed (2's comp)  n_bits=16  bin_pt=14  preci_type=Single  exp_width=8  frac_width=24  explicit_period=off  period=1  equ=P=C  opselect=C  inp2=PCIN>>17  opr=+  inp1=P  carry=CIN  dbl_ovrd=off  block_type=constant
  Constant8 : xbsIndex_r4/Constant  const=h(6,9)  gui_display_data_type=Fixed-point  arith_type=Signed (2's comp)  n_bits=16  bin_pt=14  preci_type=Single  exp_width=8  frac_width=24  explicit_period=off  period=1  equ=P=C  opselect=C  inp2=PCIN>>17  opr=+  inp1=P  carry=CIN  dbl_ovrd=off  block_type=constant
  Constant9 : xbsIndex_r4/Constant  const=h(6,8)  gui_display_data_type=Fixed-point  arith_type=Signed (2's comp)  n_bits=16  bin_pt=14  preci_type=Single  exp_width=8  frac_width=24  explicit_period=off  period=1  equ=P=C  opselect=C  inp2=PCIN>>17  opr=+  inp1=P  carry=CIN  dbl_ovrd=off  block_type=constant
  Delay{1..17} (17 alike) : xbsIndex_r4/Delay  rst=off  infoeditControl=Selection of Reset will increase slice count due to use of real FFs and instead of SRLs  en=off  latency=1  reg_retiming=off  dbl_ovrd=off  block_type=delay
  Mult{1..17} (17 alike) : xbsIndex_r4/Mult  precision=User Defined  arith_type="Signed  (2's comp)"  n_bits=16  bin_pt=14  quantization="Round  (unbiased: +/- Inf)"  overflow=Flag as error  en=off  latency=0  use_behavioral_HDL=off  opt=Speed  use_embedded=on  optimum_pipeline=off  pipeline=on  dbl_ovrd=off  use_rpm=on  placement_style=Triangular  block_type=mult
  Out1 : Outport
  wires:
  Mult2/1 -> AddSub2/2
  AddSub2/1 -> Out1/1
  Delay6/1 -> AddSub2/1
  Constant2/1 -> Mult4/1
  AddSub4/1 -> Delay1/1
  Mult4/1 -> AddSub4/2
  Delay3/1 -> AddSub4/1
  Constant4/1 -> Mult6/1
  AddSub12/1 -> Delay9/1
  Constant3/1 -> Mult3/1
  Mult13/1 -> AddSub13/2
  AddSub13/1 -> Delay16/1
  Delay7/1 -> AddSub8/1
  Constant13/1 -> Mult13/1
  Mult3/1 -> AddSub3/2
  Mult8/1 -> AddSub8/2
  Delay8/1 -> AddSub6/1
  Delay2/1 -> AddSub3/1
  AddSub3/1 -> Delay3/1
  Delay14/1 -> AddSub10/1
  AddSub11/1 -> Delay11/1
  AddSub9/1 -> Delay14/1
  AddSub6/1 -> Delay2/1
  Delay5/1 -> AddSub7/1
  Constant7/1 -> Mult7/1
  Mult5/1 -> AddSub5/2
  Constant5/1 -> Mult5/1
  Mult12/1 -> AddSub12/2
  Mult7/1 -> AddSub7/2
  AddSub7/1 -> Delay7/1
  Delay11/1 -> AddSub12/1
  Mult11/1 -> AddSub11/2
  AddSub8/1 -> Delay4/1
  Delay4/1 -> AddSub5/1
  Constant6/1 -> Mult8/1
  Mult6/1 -> AddSub6/2
  AddSub5/1 -> Delay8/1
  Delay15/1 -> AddSub16/1
  AddSub10/1 -> Delay5/1
  Delay9/1 -> AddSub9/1
  Mult10/1 -> AddSub10/2
  Delay16/1 -> AddSub14/1
  Delay13/1 -> AddSub15/1
  Mult9/1 -> AddSub9/2
  Constant8/1 -> Mult10/1
  Constant15/1 -> Mult15/1
  Constant12/1 -> Mult14/1
  Delay10/1 -> AddSub11/1
  Delay12/1 -> AddSub13/1
  AddSub16/1 -> Delay12/1
  Mult15/1 -> AddSub15/2
  AddSub14/1 -> Delay10/1
  Mult16/1 -> AddSub16/2
  Mult14/1 -> AddSub14/2
  Constant11/1 -> Mult11/1
  Constant9/1 -> Mult9/1
  AddSub15/1 -> Delay15/1
  Constant10/1 -> Mult12/1
  Constant14/1 -> Mult16/1
  In1/1 -> Delay17/1, Mult17/2, Mult15/2, Mult16/2, Mult13/2, Mult14/2, Mult11/2, Mult12/2, Mult9/2, Mult10/2, Mult7/2, Mult8/2, Mult5/2, Mult6/2, Mult3/2, Mult4/2, Mult2/2, Mult1/2
  Delay17/1 -> AddSub17/1
  AddSub17/1 -> Delay13/1
  Mult17/1 -> AddSub17/2
  Constant16/1 -> Mult17/1
  Constant/1 -> Mult2/1
  Delay1/1 -> AddSub1/1
  Mult1/1 -> AddSub1/2
  Constant1/1 -> Mult1/1
  AddSub1/1 -> Delay6/1

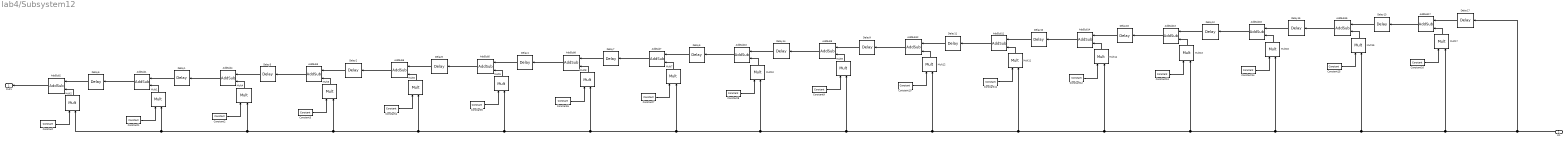
== system lab4/Subsystem12 ==
  In1 : Inport
  AddSub{1..17} (17 alike) : xbsIndex_r4/AddSub  mode=Addition  use_carryin=off  use_carryout=off  en=off  latency=0  precision=User Defined  arith_type="Signed  (2's comp)"  n_bits=17  bin_pt=14  quantization=Truncate  overflow=Wrap  use_behavioral_HDL=off  hw_selection=Fabric  pipelined=off  dbl_ovrd=off  block_type=addsub
  Constant : xbsIndex_r4/Constant  const=h(5,17)  gui_display_data_type=Fixed-point  arith_type=Signed (2's comp)  n_bits=16  bin_pt=14  preci_type=Single  exp_width=8  frac_width=24  explicit_period=off  period=1  equ=P=C  opselect=C  inp2=PCIN>>17  opr=+  inp1=P  carry=CIN  dbl_ovrd=off  block_type=constant
  Constant1 : xbsIndex_r4/Constant  const=h(5,16)  gui_display_data_type=Fixed-point  arith_type=Signed (2's comp)  n_bits=16  bin_pt=14  preci_type=Single  exp_width=8  frac_width=24  explicit_period=off  period=1  equ=P=C  opselect=C  inp2=PCIN>>17  opr=+  inp1=P  carry=CIN  dbl_ovrd=off  block_type=constant
  Constant10 : xbsIndex_r4/Constant  const=h(5,7)  gui_display_data_type=Fixed-point  arith_type=Signed (2's comp)  n_bits=16  bin_pt=14  preci_type=Single  exp_width=8  frac_width=24  explicit_period=off  period=1  equ=P=C  opselect=C  inp2=PCIN>>17  opr=+  inp1=P  carry=CIN  dbl_ovrd=off  block_type=constant
  Constant11 : xbsIndex_r4/Constant  const=h(5,6)  gui_display_data_type=Fixed-point  arith_type=Signed (2's comp)  n_bits=16  bin_pt=14  preci_type=Single  exp_width=8  frac_width=24  explicit_period=off  period=1  equ=P=C  opselect=C  inp2=PCIN>>17  opr=+  inp1=P  carry=CIN  dbl_ovrd=off  block_type=constant
  Constant12 : xbsIndex_r4/Constant  const=h(5,5)  gui_display_data_type=Fixed-point  arith_type=Signed (2's comp)  n_bits=16  bin_pt=14  preci_type=Single  exp_width=8  frac_width=24  explicit_period=off  period=1  equ=P=C  opselect=C  inp2=PCIN>>17  opr=+  inp1=P  carry=CIN  dbl_ovrd=off  block_type=constant
  Constant13 : xbsIndex_r4/Constant  const=h(5,4)  gui_display_data_type=Fixed-point  arith_type=Signed (2's comp)  n_bits=16  bin_pt=14  preci_type=Single  exp_width=8  frac_width=24  explicit_period=off  period=1  equ=P=C  opselect=C  inp2=PCIN>>17  opr=+  inp1=P  carry=CIN  dbl_ovrd=off  block_type=constant
  Constant14 : xbsIndex_r4/Constant  const=h(5,3)  gui_display_data_type=Fixed-point  arith_type=Signed (2's comp)  n_bits=16  bin_pt=14  preci_type=Single  exp_width=8  frac_width=24  explicit_period=off  period=1  equ=P=C  opselect=C  inp2=PCIN>>17  opr=+  inp1=P  carry=CIN  dbl_ovrd=off  block_type=constant
  Constant15 : xbsIndex_r4/Constant  const=h(5,2)  gui_display_data_type=Fixed-point  arith_type=Signed (2's comp)  n_bits=16  bin_pt=14  preci_type=Single  exp_width=8  frac_width=24  explicit_period=off  period=1  equ=P=C  opselect=C  inp2=PCIN>>17  opr=+  inp1=P  carry=CIN  dbl_ovrd=off  block_type=constant
  Constant16 : xbsIndex_r4/Constant  const=h(5,1)  gui_display_data_type=Fixed-point  arith_type=Signed (2's comp)  n_bits=17  bin_pt=14  preci_type=Single  exp_width=8  frac_width=24  explicit_period=off  period=1  equ=P=C  opselect=C  inp2=PCIN>>17  opr=+  inp1=P  carry=CIN  dbl_ovrd=off  block_type=constant
  Constant2 : xbsIndex_r4/Constant  const=h(5,15)  gui_display_data_type=Fixed-point  arith_type=Signed (2's comp)  n_bits=16  bin_pt=14  preci_type=Single  exp_width=8  frac_width=24  explicit_period=off  period=1  equ=P=C  opselect=C  inp2=PCIN>>17  opr=+  inp1=P  carry=CIN  dbl_ovrd=off  block_type=constant
  Constant3 : xbsIndex_r4/Constant  const=h(5,14)  gui_display_data_type=Fixed-point  arith_type=Signed (2's comp)  n_bits=16  bin_pt=14  preci_type=Single  exp_width=8  frac_width=24  explicit_period=off  period=1  equ=P=C  opselect=C  inp2=PCIN>>17  opr=+  inp1=P  carry=CIN  dbl_ovrd=off  block_type=constant
  Constant4 : xbsIndex_r4/Constant  const=h(5,13)  gui_display_data_type=Fixed-point  arith_type=Signed (2's comp)  n_bits=16  bin_pt=14  preci_type=Single  exp_width=8  frac_width=24  explicit_period=off  period=1  equ=P=C  opselect=C  inp2=PCIN>>17  opr=+  inp1=P  carry=CIN  dbl_ovrd=off  block_type=constant
  Constant5 : xbsIndex_r4/Constant  const=h(5,12)  gui_display_data_type=Fixed-point  arith_type=Signed (2's comp)  n_bits=16  bin_pt=14  preci_type=Single  exp_width=8  frac_width=24  explicit_period=off  period=1  equ=P=C  opselect=C  inp2=PCIN>>17  opr=+  inp1=P  carry=CIN  dbl_ovrd=off  block_type=constant
  Constant6 : xbsIndex_r4/Constant  const=h(5,11)  gui_display_data_type=Fixed-point  arith_type=Signed (2's comp)  n_bits=16  bin_pt=14  preci_type=Single  exp_width=8  frac_width=24  explicit_period=off  period=1  equ=P=C  opselect=C  inp2=PCIN>>17  opr=+  inp1=P  carry=CIN  dbl_ovrd=off  block_type=constant
  Constant7 : xbsIndex_r4/Constant  const=h(5,10)  gui_display_data_type=Fixed-point  arith_type=Signed (2's comp)  n_bits=16  bin_pt=14  preci_type=Single  exp_width=8  frac_width=24  explicit_period=off  period=1  equ=P=C  opselect=C  inp2=PCIN>>17  opr=+  inp1=P  carry=CIN  dbl_ovrd=off  block_type=constant
  Constant8 : xbsIndex_r4/Constant  const=h(5,9)  gui_display_data_type=Fixed-point  arith_type=Signed (2's comp)  n_bits=16  bin_pt=14  preci_type=Single  exp_width=8  frac_width=24  explicit_period=off  period=1  equ=P=C  opselect=C  inp2=PCIN>>17  opr=+  inp1=P  carry=CIN  dbl_ovrd=off  block_type=constant
  Constant9 : xbsIndex_r4/Constant  const=h(5,8)  gui_display_data_type=Fixed-point  arith_type=Signed (2's comp)  n_bits=16  bin_pt=14  preci_type=Single  exp_width=8  frac_width=24  explicit_period=off  period=1  equ=P=C  opselect=C  inp2=PCIN>>17  opr=+  inp1=P  carry=CIN  dbl_ovrd=off  block_type=constant
  Delay{1..17} (17 alike) : xbsIndex_r4/Delay  rst=off  infoeditControl=Selection of Reset will increase slice count due to use of real FFs and instead of SRLs  en=off  latency=1  reg_retiming=off  dbl_ovrd=off  block_type=delay
  Mult{1..17} (17 alike) : xbsIndex_r4/Mult  precision=User Defined  arith_type="Signed  (2's comp)"  n_bits=16  bin_pt=14  quantization="Round  (unbiased: +/- Inf)"  overflow=Flag as error  en=off  latency=0  use_behavioral_HDL=off  opt=Speed  use_embedded=on  optimum_pipeline=off  pipeline=on  dbl_ovrd=off  use_rpm=on  placement_style=Triangular  block_type=mult
  Out1 : Outport
  wires:
  Mult2/1 -> AddSub2/2
  AddSub2/1 -> Out1/1
  Delay6/1 -> AddSub2/1
  Constant2/1 -> Mult4/1
  AddSub4/1 -> Delay1/1
  Mult4/1 -> AddSub4/2
  Delay3/1 -> AddSub4/1
  Constant4/1 -> Mult6/1
  AddSub12/1 -> Delay9/1
  Constant3/1 -> Mult3/1
  Mult13/1 -> AddSub13/2
  AddSub13/1 -> Delay16/1
  Delay7/1 -> AddSub8/1
  Constant13/1 -> Mult13/1
  Mult3/1 -> AddSub3/2
  Mult8/1 -> AddSub8/2
  Delay8/1 -> AddSub6/1
  Delay2/1 -> AddSub3/1
  AddSub3/1 -> Delay3/1
  Delay14/1 -> AddSub10/1
  AddSub11/1 -> Delay11/1
  AddSub9/1 -> Delay14/1
  AddSub6/1 -> Delay2/1
  Delay5/1 -> AddSub7/1
  Constant7/1 -> Mult7/1
  Mult5/1 -> AddSub5/2
  Constant5/1 -> Mult5/1
  Mult12/1 -> AddSub12/2
  Mult7/1 -> AddSub7/2
  AddSub7/1 -> Delay7/1
  Delay11/1 -> AddSub12/1
  Mult11/1 -> AddSub11/2
  AddSub8/1 -> Delay4/1
  Delay4/1 -> AddSub5/1
  Constant6/1 -> Mult8/1
  Mult6/1 -> AddSub6/2
  AddSub5/1 -> Delay8/1
  Delay15/1 -> AddSub16/1
  AddSub10/1 -> Delay5/1
  Delay9/1 -> AddSub9/1
  Mult10/1 -> AddSub10/2
  Delay16/1 -> AddSub14/1
  Delay13/1 -> AddSub15/1
  Mult9/1 -> AddSub9/2
  Constant8/1 -> Mult10/1
  Constant15/1 -> Mult15/1
  Constant12/1 -> Mult14/1
  Delay10/1 -> AddSub11/1
  Delay12/1 -> AddSub13/1
  AddSub16/1 -> Delay12/1
  Mult15/1 -> AddSub15/2
  AddSub14/1 -> Delay10/1
  Mult16/1 -> AddSub16/2
  Mult14/1 -> AddSub14/2
  Constant11/1 -> Mult11/1
  Constant9/1 -> Mult9/1
  AddSub15/1 -> Delay15/1
  Constant10/1 -> Mult12/1
  Constant14/1 -> Mult16/1
  In1/1 -> Delay17/1, Mult17/2, Mult15/2, Mult16/2, Mult13/2, Mult14/2, Mult11/2, Mult12/2, Mult9/2, Mult10/2, Mult7/2, Mult8/2, Mult5/2, Mult6/2, Mult3/2, Mult4/2, Mult2/2, Mult1/2
  Delay17/1 -> AddSub17/1
  AddSub17/1 -> Delay13/1
  Mult17/1 -> AddSub17/2
  Constant16/1 -> Mult17/1
  Constant/1 -> Mult2/1
  Delay1/1 -> AddSub1/1
  Mult1/1 -> AddSub1/2
  Constant1/1 -> Mult1/1
  AddSub1/1 -> Delay6/1
